simulink model "final"  (R2022b)
settings: Solver=VariableStepAuto  StartTime=0.0  StopTime=35  MaxStep=1e-4  RelTol=1e-3
libraries: simulink x8, slpidlib x5
settings Model: Creator=marco  LastModifiedBy=marco
settings SolverCC: ZeroCrossAlgorithm=Adaptive
settings DebuggingCC: MaskedZcDiagnostic=none  IgnoredZcDiagnostic=none

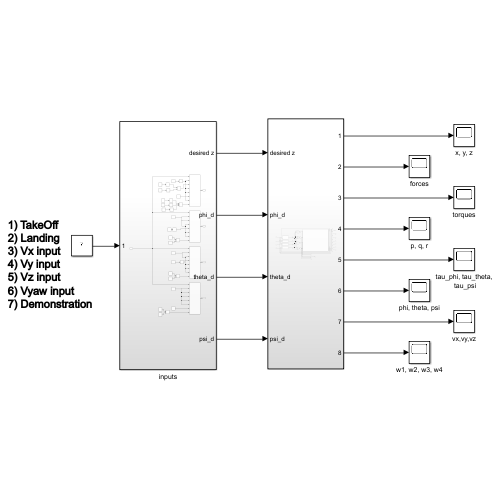
[thumbnail: Simulink's stored preview of the top-level diagram]
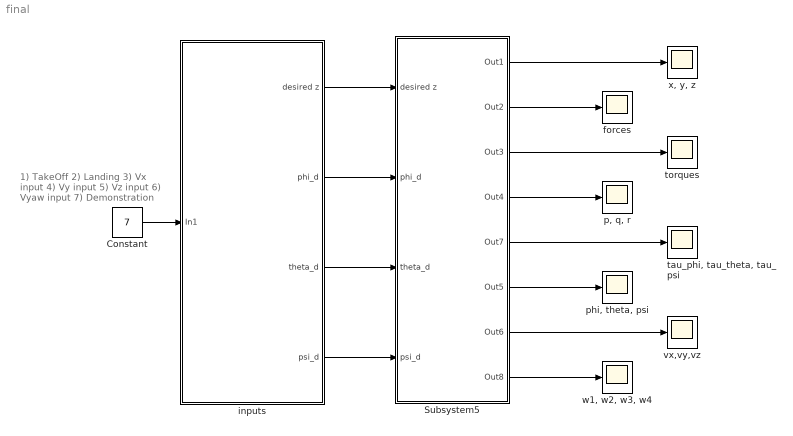
== system final ==
  note: 1) TakeOff
      | 2) Landing
      | 3) Vx input
      | 4) Vy input
      | 5) Vz input
      | 6) Vyaw input
      | 7) Demonstration
  Constant : Constant  Value=7
  Subsystem5 : Subsystem
  forces : Scope
  inputs : Subsystem
  "p, q, r" : Scope
  "phi, theta, psi" : Scope
  "tau_phi, tau_theta, tau_psi" : Scope
  torques : Scope
  vx,vy,vz : Scope
  "w1, w2, w3, w4" : Scope
  "x, y, z" : Scope
  wires:
  Constant/1 -> inputs/1(In1)
  inputs/1(desired z) -> Subsystem5/1(desired z)
  inputs/2(phi_d) -> Subsystem5/2(phi_d)
  inputs/3(theta_d) -> Subsystem5/3(theta_d)
  inputs/4(psi_d) -> Subsystem5/4(psi_d)
  Subsystem5/1(Out1) -> "x, y, z"/1
  Subsystem5/2(Out2) -> forces/1
  Subsystem5/3(Out3) -> torques/1
  Subsystem5/4(Out4) -> "p, q, r"/1
  Subsystem5/6(Out5) -> "phi, theta, psi"/1
  Subsystem5/7(Out6) -> vx,vy,vz/1
  Subsystem5/5(Out7) -> "tau_phi, tau_theta, tau_psi"/1
  Subsystem5/8(Out8) -> "w1, w2, w3, w4"/1

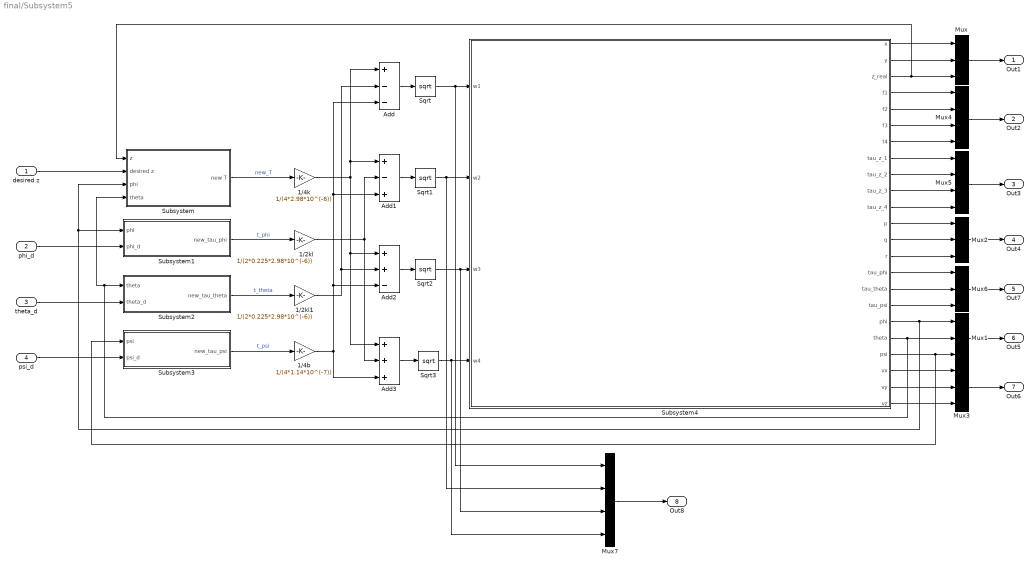
== system final/Subsystem5 ==
  desired z : Inport
  phi_d : Inport  Port=2
  theta_d : Inport  Port=3
  psi_d : Inport  Port=4
  1/2kl : Gain  Gain=1/(2*0.225*2.98*10^(-6))
  1/2kl1 : Gain  Gain=1/(2*0.225*2.98*10^(-6))
  1/4b : Gain  Gain=1/(4*1.14*10^(-7))
  1/4k : Gain  Gain=1/(4*2.98*10^(-6))
  Add : Sum  Inputs=+--
  Add1 : Sum  Inputs=+-+
  Add2 : Sum  Inputs=++-
  Add3 : Sum  Inputs=+++
  Mux{,1..3,6} (5 alike) : Mux  Inputs=3
  Mux4 : Mux
  Mux5 : Mux
  Mux7 : Mux
  Sqrt{,1..3} (4 alike) : Sqrt
  Subsystem : Subsystem
  Subsystem1 : Subsystem
  Subsystem2 : Subsystem
  Subsystem3 : Subsystem
  Subsystem4 : Subsystem
  Out1 : Outport
  Out2 : Outport  Port=2
  Out3 : Outport  Port=3
  Out4 : Outport  Port=4
  Out7 : Outport  Port=5
  Out5 : Outport  Port=6
  Out6 : Outport  Port=7
  Out8 : Outport  Port=8
  wires:
  Subsystem4/3(z_real) -> Subsystem/1(z), Mux/3
  Subsystem4/8(tau_z_1) -> Mux5/1
  1/4k/1 -> Add3/1, Add2/1, Add1/1, Add/1
  Subsystem4/19(theta) -> Subsystem2/1(theta), Subsystem/4(theta), Mux1/2
  Subsystem4/6(f3) -> Mux4/3
  Subsystem4/1(x) -> Mux/1
  Sqrt/1 -> Mux7/1, Subsystem4/1(w1)
  Mux4/1 -> Out2/1
  Subsystem4/20(psi) -> Subsystem3/1(psi), Mux1/3
  Subsystem4/4(f1) -> Mux4/1
  Subsystem4/15(tau_phi) -> Mux6/1
  1/2kl1/1 -> Add2/2, Add/2
  Subsystem4/17(tau_psi) -> Mux6/3
  Subsystem4/10(tau_z_3) -> Mux5/3
  Subsystem4/18(phi) -> Subsystem1/1(phi), Subsystem/3(phi), Mux1/1
  Subsystem4/16(tau_theta) -> Mux6/2
  Subsystem4/21(vx) -> Mux3/1
  Subsystem4/5(f2) -> Mux4/2
  Subsystem4/7(f4) -> Mux4/4
  Subsystem4/22(vy) -> Mux3/2
  Add1/1 -> Sqrt1/1
  Subsystem4/11(tau_z_4) -> Mux5/4
  Mux/1 -> Out1/1
  Sqrt1/1 -> Mux7/2, Subsystem4/2(w2)
  Mux6/1 -> Out7/1
  Subsystem3/1(new_tau_psi) -> 1/4b/1  "t_psi"
  Subsystem4/9(tau_z_2) -> Mux5/2
  1/4b/1 -> Add3/3, Add2/3, Add1/3, Add/3
  theta_d/1 -> Subsystem2/2(theta_d)
  Subsystem4/14(r) -> Mux2/3
  Subsystem/1(new T) -> 1/4k/1  "new_T"
  Subsystem2/1(new_tau_theta) -> 1/2kl1/1  "t_theta"
  Mux2/1 -> Out4/1
  Add3/1 -> Sqrt3/1
  Subsystem4/13(q) -> Mux2/2
  Subsystem4/12(p) -> Mux2/1
  Subsystem4/2(y) -> Mux/2
  1/2kl/1 -> Add3/2, Add1/2
  Sqrt3/1 -> Mux7/4, Subsystem4/4(w4)
  phi_d/1 -> Subsystem1/2(phi_d)
  Sqrt2/1 -> Mux7/3, Subsystem4/3(w3)
  Subsystem1/1(new_tau_phi) -> 1/2kl/1  "t_phi"
  Subsystem4/23(vz) -> Mux3/3
  Mux1/1 -> Out5/1
  Add2/1 -> Sqrt2/1
  Add/1 -> Sqrt/1
  Mux5/1 -> Out3/1
  desired z/1 -> Subsystem/2(desired z)
  Mux3/1 -> Out6/1
  psi_d/1 -> Subsystem3/2(psi_d)
  Mux7/1 -> Out8/1

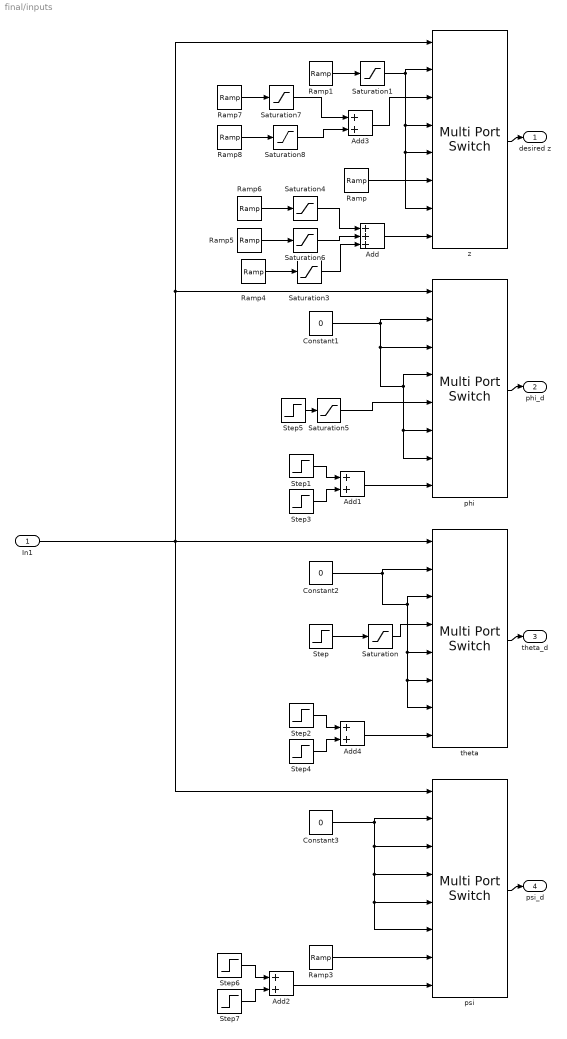
== system final/inputs ==
  In1 : Inport
  Add : Sum  Inputs=+++
  Add{1..4} (4 alike) : Sum
  Constant1 : Constant  Value=0
  Constant2 : Constant  Value=0
  Constant3 : Constant  Value=0
  Ramp : simulink/Sources/Ramp  slope=2  start=0  InitialOutput=0
  Ramp1 : simulink/Sources/Ramp  slope=1  start=0  InitialOutput=0
  Ramp3 : simulink/Sources/Ramp  slope=1  start=0  InitialOutput=0
  Ramp4 : simulink/Sources/Ramp  slope=-1  start=30  InitialOutput=0
  Ramp5 : simulink/Sources/Ramp  slope=1  start=25  InitialOutput=0
  Ramp6 : simulink/Sources/Ramp  slope=2.5  start=0  InitialOutput=0
  Ramp7 : simulink/Sources/Ramp  slope=1  start=0  InitialOutput=0
  Ramp8 : simulink/Sources/Ramp  slope=-1  start=5  InitialOutput=0
  Saturation : Saturate  UpperLimit=0.2
  Saturation{1,4,6..7} (4 alike) : Saturate  UpperLimit=1
  Saturation3 : Saturate  UpperLimit=inf  LowerLimit=-2
  Saturation5 : Saturate  UpperLimit=inf  LowerLimit=-9
  Saturation8 : Saturate  UpperLimit=1  LowerLimit=-1
  Step : Step  Time=7  After=0.05  SampleTime=0
  Step1 : Step  Time=15  After=-0.051  SampleTime=0
  Step2 : Step  Time=5  After=0.051  SampleTime=0
  Step3 : Step  Time=16  After=0.051  SampleTime=0
  Step4 : Step  Time=6  After=-0.051  SampleTime=0
  Step5 : Step  Time=5  After=-0.2  SampleTime=0
  Step6 : Step  Time=25  After=0.05  SampleTime=0
  Step7 : Step  Time=26  After=-0.05  SampleTime=0
  phi : MultiPortSwitch  Inputs=7  SaturateOnIntegerOverflow=off  InputSameDT=off
  psi : MultiPortSwitch  Inputs=7  SaturateOnIntegerOverflow=off  InputSameDT=off
  theta : MultiPortSwitch  Inputs=7  SaturateOnIntegerOverflow=off  InputSameDT=off
  z : MultiPortSwitch  Inputs=7  SaturateOnIntegerOverflow=off  InputSameDT=off
  desired z : Outport
  phi_d : Outport  Port=2
  theta_d : Outport  Port=3
  psi_d : Outport  Port=4
  wires:
  Constant2/1 -> theta/7, theta/6, theta/5, theta/3, theta/2
  Step/1 -> Saturation/1
  Constant1/1 -> phi/7, phi/6, phi/4, phi/3, phi/2
  Ramp/1 -> z/6
  Saturation1/1 -> z/7, z/5, z/4, z/2
  Constant3/1 -> psi/6, psi/5, psi/4, psi/3, psi/2
  In1/1 -> phi/1, z/1, psi/1, theta/1
  theta/1 -> theta_d/1
  Saturation/1 -> theta/4
  Ramp3/1 -> psi/7
  Ramp1/1 -> Saturation1/1
  Step5/1 -> Saturation5/1
  phi/1 -> phi_d/1
  z/1 -> desired z/1
  psi/1 -> psi_d/1
  Step4/1 -> Add4/2
  Step2/1 -> Add4/1
  Add4/1 -> theta/8
  Saturation5/1 -> phi/5
  Step1/1 -> Add1/1
  Step3/1 -> Add1/2
  Add1/1 -> phi/8
  Step6/1 -> Add2/1
  Step7/1 -> Add2/2
  Add2/1 -> psi/8
  Ramp5/1 -> Saturation6/1
  Saturation4/1 -> Add/1
  Saturation6/1 -> Add/2
  Ramp6/1 -> Saturation4/1
  Ramp4/1 -> Saturation3/1
  Saturation3/1 -> Add/3
  Add/1 -> z/8
  Saturation7/1 -> Add3/1
  Saturation8/1 -> Add3/2
  Ramp8/1 -> Saturation8/1
  Add3/1 -> z/3
  Ramp7/1 -> Saturation7/1

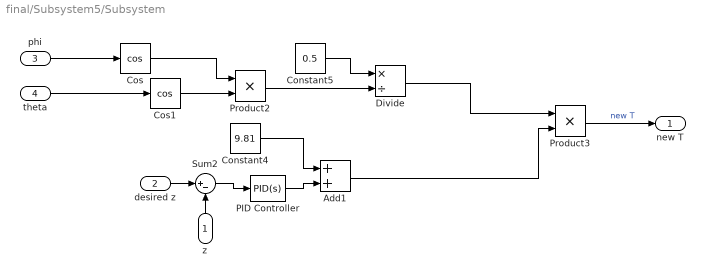
== system final/Subsystem5/Subsystem ==
  z : Inport
  desired z : Inport  Port=2
  phi : Inport  Port=3
  theta : Inport  Port=4
  Add1 : Sum
  Constant4 : Constant  Value=9.81
  Constant5 : Constant  Value=0.5
  Cos : Trigonometry  Operator=cos
  Cos1 : Trigonometry  Operator=cos
  Divide : Product  Inputs=*/
  PID Controller : slpidlib/PID Controller  Controller=PID  Form=Parallel  TimeDomain=Continuous-time  UseExternalTs=off  SampleTime=-1  IntegratorMethod=Forward Euler  FilterMethod=Forward Euler  ControllerParametersSource=internal  P=7.12587279082995  I=2.27236958573159  UseKiTs=off  D=5.19851443495758  N=56.2861343217854  UseFilter=on  TunerSelectOption=Transfer Function Based (PID Tuner App)  InitialConditionSource=internal  InitialConditionForIntegrator=0  InitialConditionForFilter=0  DifferentiatorICPrevScaledInput=0  ExternalReset=none  TrackingMode=off  Kt=1  LimitOutput=off  SatLimitsSource=internal  UpperSaturationLimit=inf  LowerSaturationLimit=-inf  LinearizeAsGain=on  AntiWindupMode=none  Kb=1  LimitIntegrator=off  UpperIntegratorSaturationLimit=inf  LowerIntegratorSaturationLimit=-inf  POutMin=[]  POutMax=[]  IOutMin=[]  IOutMax=[]  DOutMin=[]  DOutMax=[]  NOutMin=[]  NOutMax=[]  SumOutMin=[]  SumOutMax=[]  SaturationOutMin=[]  SaturationOutMax=[]  PParamMin=[]  PParamMax=[]  IParamMin=[]  IParamMax=[]  DParamMin=[]  DParamMax=[]  NParamMin=[]  NParamMax=[]  KbParamMin=[]  KbParamMax=[]  KtParamMin=[]  KtParamMax=[]  KbOutMin=[]  KbOutMax=[]  KtOutMin=[]  KtOutMax=[]  IntegratorOutMin=[]  IntegratorOutMax=[]  FilterOutMin=[]  FilterOutMax=[]  SumI1OutMin=[]  SumI1OutMax=[]  SumI2OutMin=[]  SumI2OutMax=[]  SumI3OutMin=[]  SumI3OutMax=[]  SumI4OutMin=[]  SumI4OutMax=[]  SumDOutMin=[]  SumDOutMax=[]  DifferentiatorOutMin=[]  DifferentiatorOutMax=[]  FilterDiffOutCoefMin=[]  FilterDiffOutCoefMax=[]  ReciprocalOutMin=[]  ReciprocalOutMax=[]  SumDenOutMin=[]  SumDenOutMax=[]  SumNumOutMin=[]  SumNumOutMax=[]  DivideOutMin=[]  DivideOutMax=[]  UdiffTsProdOutMin=[]  UdiffTsProdOutMax=[]  NTsProdOutMin=[]  NTsProdOutMax=[]  UintegralTsProdOutMin=[]  UintegralTsProdOutMax=[]  UngainTsProdOutMin=[]  UngainTsProdOutMax=[]  ClampingZeroOutDataTypeStr=Inherit: Inherit via back propagation  ClampingZeroOutMin=[]  ClampingZeroOutMax=[]  FilterDenConstantOutDataTypeStr=Inherit: Inherit via back propagation  FilterDenConstantOutMin=[]  FilterDenConstantOutMax=[]  PCopyOutDataTypeStr=Inherit: Inherit via back propagation  PCopyOutMin=[]  PCopyOutMax=[]  NCopyOutDataTypeStr=Inherit: Inherit via back propagation  NCopyOutMin=[]  NCopyOutMax=[]  IntegratorContinuousStateAttributes=''  IntegratorStateMustResolveToSignalObject=off  IntegratorRTWStateStorageClass=Auto  FilterContinuousStateAttributes=''  FilterStateMustResolveToSignalObject=off  FilterRTWStateStorageClass=Auto  ParallelPVariant=InternalParameters  IdealPVariant=Disabled  IVariant=InternalParameters  DVariant=InternalParameters  IntegratorVariant=Continuous  SatVariant=Disabled  AWVariant=Passthrough  PCopyVariant=Disabled  TRVariant=Disabled  FdbkBlocksVariant=Forward  IdealPFdbkVariant=Disabled  SatFdbkVariant=Disabled  DerivativeFilterVariant=ContFilter  NVariant=InternalParameters  NCopyVariant=Disabled  FilterICVariant=InternalICsFilter  IntegratorICVariant=InternalICs  ExternalResetVariant=Disabled  TRSumVariant=Passthrough  SumFdbkVariant=Disabled  SumVariant=Sum_PID  TsampFilterVariant=InternalTs  TsampNgainVariant=Passthrough  TsampIntegralVariant=Passthrough  ExternalSaturationOutDataTypeStr=Inherit: Same as second input
  Product2 : Product
  Product3 : Product
  Sum2 : Sum  Inputs=|+-
  new T : Outport
  wires:
  Constant4/1 -> Add1/1
  Product2/1 -> Divide/2
  Divide/1 -> Product3/1
  Product3/1 -> new T/1  "new T"
  Cos/1 -> Product2/1
  phi/1 -> Cos/1
  Cos1/1 -> Product2/2
  z/1 -> Sum2/2
  Constant5/1 -> Divide/1
  theta/1 -> Cos1/1
  desired z/1 -> Sum2/1
  Sum2/1 -> PID Controller/1
  PID Controller/1 -> Add1/2
  Add1/1 -> Product3/2

== system final/Subsystem5/Subsystem1 ==
  phi : Inport
  phi_d : Inport  Port=2
  Ix : Gain  Gain=4.856*10^(-3)
  PID Controller : slpidlib/PID Controller  Controller=PID  Form=Parallel  TimeDomain=Continuous-time  UseExternalTs=off  SampleTime=-1  IntegratorMethod=Forward Euler  FilterMethod=Forward Euler  ControllerParametersSource=internal  P=7.44259083470397  I=2.2059084504827  UseKiTs=off  D=6.16600811387227  N=34.5297262058638  UseFilter=on  TunerSelectOption=Transfer Function Based (PID Tuner App)  InitialConditionSource=internal  InitialConditionForIntegrator=0  InitialConditionForFilter=0  DifferentiatorICPrevScaledInput=0  ExternalReset=none  TrackingMode=off  Kt=1  LimitOutput=off  SatLimitsSource=internal  UpperSaturationLimit=inf  LowerSaturationLimit=-inf  LinearizeAsGain=on  AntiWindupMode=none  Kb=1  LimitIntegrator=off  UpperIntegratorSaturationLimit=inf  LowerIntegratorSaturationLimit=-inf  POutMin=[]  POutMax=[]  IOutMin=[]  IOutMax=[]  DOutMin=[]  DOutMax=[]  NOutMin=[]  NOutMax=[]  SumOutMin=[]  SumOutMax=[]  SaturationOutMin=[]  SaturationOutMax=[]  PParamMin=[]  PParamMax=[]  IParamMin=[]  IParamMax=[]  DParamMin=[]  DParamMax=[]  NParamMin=[]  NParamMax=[]  KbParamMin=[]  KbParamMax=[]  KtParamMin=[]  KtParamMax=[]  KbOutMin=[]  KbOutMax=[]  KtOutMin=[]  KtOutMax=[]  IntegratorOutMin=[]  IntegratorOutMax=[]  FilterOutMin=[]  FilterOutMax=[]  SumI1OutMin=[]  SumI1OutMax=[]  SumI2OutMin=[]  SumI2OutMax=[]  SumI3OutMin=[]  SumI3OutMax=[]  SumI4OutMin=[]  SumI4OutMax=[]  SumDOutMin=[]  SumDOutMax=[]  DifferentiatorOutMin=[]  DifferentiatorOutMax=[]  FilterDiffOutCoefMin=[]  FilterDiffOutCoefMax=[]  ReciprocalOutMin=[]  ReciprocalOutMax=[]  SumDenOutMin=[]  SumDenOutMax=[]  SumNumOutMin=[]  SumNumOutMax=[]  DivideOutMin=[]  DivideOutMax=[]  UdiffTsProdOutMin=[]  UdiffTsProdOutMax=[]  NTsProdOutMin=[]  NTsProdOutMax=[]  UintegralTsProdOutMin=[]  UintegralTsProdOutMax=[]  UngainTsProdOutMin=[]  UngainTsProdOutMax=[]  ClampingZeroOutDataTypeStr=Inherit: Inherit via back propagation  ClampingZeroOutMin=[]  ClampingZeroOutMax=[]  FilterDenConstantOutDataTypeStr=Inherit: Inherit via back propagation  FilterDenConstantOutMin=[]  FilterDenConstantOutMax=[]  PCopyOutDataTypeStr=Inherit: Inherit via back propagation  PCopyOutMin=[]  PCopyOutMax=[]  NCopyOutDataTypeStr=Inherit: Inherit via back propagation  NCopyOutMin=[]  NCopyOutMax=[]  IntegratorContinuousStateAttributes=''  IntegratorStateMustResolveToSignalObject=off  IntegratorRTWStateStorageClass=Auto  FilterContinuousStateAttributes=''  FilterStateMustResolveToSignalObject=off  FilterRTWStateStorageClass=Auto  ParallelPVariant=InternalParameters  IdealPVariant=Disabled  IVariant=InternalParameters  DVariant=InternalParameters  IntegratorVariant=Continuous  SatVariant=Disabled  AWVariant=Passthrough  PCopyVariant=Disabled  TRVariant=Disabled  FdbkBlocksVariant=Forward  IdealPFdbkVariant=Disabled  SatFdbkVariant=Disabled  DerivativeFilterVariant=ContFilter  NVariant=InternalParameters  NCopyVariant=Disabled  FilterICVariant=InternalICsFilter  IntegratorICVariant=InternalICs  ExternalResetVariant=Disabled  TRSumVariant=Passthrough  SumFdbkVariant=Disabled  SumVariant=Sum_PID  TsampFilterVariant=InternalTs  TsampNgainVariant=Passthrough  TsampIntegralVariant=Passthrough  ExternalSaturationOutDataTypeStr=Inherit: Same as second input
  Sum2 : Sum  Inputs=|+-
  new_tau_phi : Outport
  wires:
  phi_d/1 -> Sum2/1
  phi/1 -> Sum2/2
  Ix/1 -> new_tau_phi/1
  Sum2/1 -> PID Controller/1
  PID Controller/1 -> Ix/1

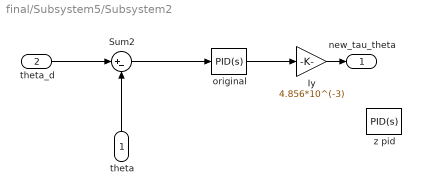
== system final/Subsystem5/Subsystem2 ==
  theta : Inport
  theta_d : Inport  Port=2
  Iy : Gain  Gain=4.856*10^(-3)
  Sum2 : Sum  Inputs=|+-
  original : slpidlib/PID Controller  Controller=PID  Form=Parallel  TimeDomain=Continuous-time  UseExternalTs=off  SampleTime=-1  IntegratorMethod=Forward Euler  FilterMethod=Forward Euler  ControllerParametersSource=internal  P=7.44259083470397  I=2.2059084504827  UseKiTs=off  D=6.16600811387227  N=34.5297262058638  UseFilter=on  TunerSelectOption=Transfer Function Based (PID Tuner App)  InitialConditionSource=internal  InitialConditionForIntegrator=0  InitialConditionForFilter=0  DifferentiatorICPrevScaledInput=0  ExternalReset=none  TrackingMode=off  Kt=1  LimitOutput=off  SatLimitsSource=internal  UpperSaturationLimit=inf  LowerSaturationLimit=-inf  LinearizeAsGain=on  AntiWindupMode=none  Kb=1  LimitIntegrator=off  UpperIntegratorSaturationLimit=inf  LowerIntegratorSaturationLimit=-inf  POutMin=[]  POutMax=[]  IOutMin=[]  IOutMax=[]  DOutMin=[]  DOutMax=[]  NOutMin=[]  NOutMax=[]  SumOutMin=[]  SumOutMax=[]  SaturationOutMin=[]  SaturationOutMax=[]  PParamMin=[]  PParamMax=[]  IParamMin=[]  IParamMax=[]  DParamMin=[]  DParamMax=[]  NParamMin=[]  NParamMax=[]  KbParamMin=[]  KbParamMax=[]  KtParamMin=[]  KtParamMax=[]  KbOutMin=[]  KbOutMax=[]  KtOutMin=[]  KtOutMax=[]  IntegratorOutMin=[]  IntegratorOutMax=[]  FilterOutMin=[]  FilterOutMax=[]  SumI1OutMin=[]  SumI1OutMax=[]  SumI2OutMin=[]  SumI2OutMax=[]  SumI3OutMin=[]  SumI3OutMax=[]  SumI4OutMin=[]  SumI4OutMax=[]  SumDOutMin=[]  SumDOutMax=[]  DifferentiatorOutMin=[]  DifferentiatorOutMax=[]  FilterDiffOutCoefMin=[]  FilterDiffOutCoefMax=[]  ReciprocalOutMin=[]  ReciprocalOutMax=[]  SumDenOutMin=[]  SumDenOutMax=[]  SumNumOutMin=[]  SumNumOutMax=[]  DivideOutMin=[]  DivideOutMax=[]  UdiffTsProdOutMin=[]  UdiffTsProdOutMax=[]  NTsProdOutMin=[]  NTsProdOutMax=[]  UintegralTsProdOutMin=[]  UintegralTsProdOutMax=[]  UngainTsProdOutMin=[]  UngainTsProdOutMax=[]  ClampingZeroOutDataTypeStr=Inherit: Inherit via back propagation  ClampingZeroOutMin=[]  ClampingZeroOutMax=[]  FilterDenConstantOutDataTypeStr=Inherit: Inherit via back propagation  FilterDenConstantOutMin=[]  FilterDenConstantOutMax=[]  PCopyOutDataTypeStr=Inherit: Inherit via back propagation  PCopyOutMin=[]  PCopyOutMax=[]  NCopyOutDataTypeStr=Inherit: Inherit via back propagation  NCopyOutMin=[]  NCopyOutMax=[]  IntegratorContinuousStateAttributes=''  IntegratorStateMustResolveToSignalObject=off  IntegratorRTWStateStorageClass=Auto  FilterContinuousStateAttributes=''  FilterStateMustResolveToSignalObject=off  FilterRTWStateStorageClass=Auto  ParallelPVariant=InternalParameters  IdealPVariant=Disabled  IVariant=InternalParameters  DVariant=InternalParameters  IntegratorVariant=Continuous  SatVariant=Disabled  AWVariant=Passthrough  PCopyVariant=Disabled  TRVariant=Disabled  FdbkBlocksVariant=Forward  IdealPFdbkVariant=Disabled  SatFdbkVariant=Disabled  DerivativeFilterVariant=ContFilter  NVariant=InternalParameters  NCopyVariant=Disabled  FilterICVariant=InternalICsFilter  IntegratorICVariant=InternalICs  ExternalResetVariant=Disabled  TRSumVariant=Passthrough  SumFdbkVariant=Disabled  SumVariant=Sum_PID  TsampFilterVariant=InternalTs  TsampNgainVariant=Passthrough  TsampIntegralVariant=Passthrough  ExternalSaturationOutDataTypeStr=Inherit: Same as second input
  z pid : slpidlib/PID Controller  Controller=PID  Form=Parallel  TimeDomain=Continuous-time  UseExternalTs=off  SampleTime=-1  IntegratorMethod=Forward Euler  FilterMethod=Forward Euler  ControllerParametersSource=internal  P=7.12587279082995  I=2.27236958573159  UseKiTs=off  D=5.19851443495758  N=56.2861343217854  UseFilter=on  TunerSelectOption=Transfer Function Based (PID Tuner App)  InitialConditionSource=internal  InitialConditionForIntegrator=0  InitialConditionForFilter=0  DifferentiatorICPrevScaledInput=0  ExternalReset=none  TrackingMode=off  Kt=1  LimitOutput=off  SatLimitsSource=internal  UpperSaturationLimit=inf  LowerSaturationLimit=-inf  LinearizeAsGain=on  AntiWindupMode=none  Kb=1  LimitIntegrator=off  UpperIntegratorSaturationLimit=inf  LowerIntegratorSaturationLimit=-inf  POutMin=[]  POutMax=[]  IOutMin=[]  IOutMax=[]  DOutMin=[]  DOutMax=[]  NOutMin=[]  NOutMax=[]  SumOutMin=[]  SumOutMax=[]  SaturationOutMin=[]  SaturationOutMax=[]  PParamMin=[]  PParamMax=[]  IParamMin=[]  IParamMax=[]  DParamMin=[]  DParamMax=[]  NParamMin=[]  NParamMax=[]  KbParamMin=[]  KbParamMax=[]  KtParamMin=[]  KtParamMax=[]  KbOutMin=[]  KbOutMax=[]  KtOutMin=[]  KtOutMax=[]  IntegratorOutMin=[]  IntegratorOutMax=[]  FilterOutMin=[]  FilterOutMax=[]  SumI1OutMin=[]  SumI1OutMax=[]  SumI2OutMin=[]  SumI2OutMax=[]  SumI3OutMin=[]  SumI3OutMax=[]  SumI4OutMin=[]  SumI4OutMax=[]  SumDOutMin=[]  SumDOutMax=[]  DifferentiatorOutMin=[]  DifferentiatorOutMax=[]  FilterDiffOutCoefMin=[]  FilterDiffOutCoefMax=[]  ReciprocalOutMin=[]  ReciprocalOutMax=[]  SumDenOutMin=[]  SumDenOutMax=[]  SumNumOutMin=[]  SumNumOutMax=[]  DivideOutMin=[]  DivideOutMax=[]  UdiffTsProdOutMin=[]  UdiffTsProdOutMax=[]  NTsProdOutMin=[]  NTsProdOutMax=[]  UintegralTsProdOutMin=[]  UintegralTsProdOutMax=[]  UngainTsProdOutMin=[]  UngainTsProdOutMax=[]  ClampingZeroOutDataTypeStr=Inherit: Inherit via back propagation  ClampingZeroOutMin=[]  ClampingZeroOutMax=[]  FilterDenConstantOutDataTypeStr=Inherit: Inherit via back propagation  FilterDenConstantOutMin=[]  FilterDenConstantOutMax=[]  PCopyOutDataTypeStr=Inherit: Inherit via back propagation  PCopyOutMin=[]  PCopyOutMax=[]  NCopyOutDataTypeStr=Inherit: Inherit via back propagation  NCopyOutMin=[]  NCopyOutMax=[]  IntegratorContinuousStateAttributes=''  IntegratorStateMustResolveToSignalObject=off  IntegratorRTWStateStorageClass=Auto  FilterContinuousStateAttributes=''  FilterStateMustResolveToSignalObject=off  FilterRTWStateStorageClass=Auto  ParallelPVariant=InternalParameters  IdealPVariant=Disabled  IVariant=InternalParameters  DVariant=InternalParameters  IntegratorVariant=Continuous  SatVariant=Disabled  AWVariant=Passthrough  PCopyVariant=Disabled  TRVariant=Disabled  FdbkBlocksVariant=Forward  IdealPFdbkVariant=Disabled  SatFdbkVariant=Disabled  DerivativeFilterVariant=ContFilter  NVariant=InternalParameters  NCopyVariant=Disabled  FilterICVariant=InternalICsFilter  IntegratorICVariant=InternalICs  ExternalResetVariant=Disabled  TRSumVariant=Passthrough  SumFdbkVariant=Disabled  SumVariant=Sum_PID  TsampFilterVariant=InternalTs  TsampNgainVariant=Passthrough  TsampIntegralVariant=Passthrough  ExternalSaturationOutDataTypeStr=Inherit: Same as second input
  new_tau_theta : Outport
  wires:
  theta_d/1 -> Sum2/1
  theta/1 -> Sum2/2
  Iy/1 -> new_tau_theta/1
  original/1 -> Iy/1
  Sum2/1 -> original/1

== system final/Subsystem5/Subsystem3 ==
  psi : Inport
  psi_d : Inport  Port=2
  Iz : Gain  Gain=8.801*10^(-3)
  PID Controller1 : slpidlib/PID Controller  Controller=PID  Form=Parallel  TimeDomain=Continuous-time  UseExternalTs=off  SampleTime=-1  IntegratorMethod=Forward Euler  FilterMethod=Forward Euler  ControllerParametersSource=internal  P=19.126699464281  I=9.13192175933972  UseKiTs=off  D=9.75332765558192  N=36.46824066771  UseFilter=on  TunerSelectOption=Transfer Function Based (PID Tuner App)  InitialConditionSource=internal  InitialConditionForIntegrator=0  InitialConditionForFilter=0  DifferentiatorICPrevScaledInput=0  ExternalReset=none  TrackingMode=off  Kt=1  LimitOutput=off  SatLimitsSource=internal  UpperSaturationLimit=inf  LowerSaturationLimit=-inf  LinearizeAsGain=on  AntiWindupMode=none  Kb=1  LimitIntegrator=off  UpperIntegratorSaturationLimit=inf  LowerIntegratorSaturationLimit=-inf  POutMin=[]  POutMax=[]  IOutMin=[]  IOutMax=[]  DOutMin=[]  DOutMax=[]  NOutMin=[]  NOutMax=[]  SumOutMin=[]  SumOutMax=[]  SaturationOutMin=[]  SaturationOutMax=[]  PParamMin=[]  PParamMax=[]  IParamMin=[]  IParamMax=[]  DParamMin=[]  DParamMax=[]  NParamMin=[]  NParamMax=[]  KbParamMin=[]  KbParamMax=[]  KtParamMin=[]  KtParamMax=[]  KbOutMin=[]  KbOutMax=[]  KtOutMin=[]  KtOutMax=[]  IntegratorOutMin=[]  IntegratorOutMax=[]  FilterOutMin=[]  FilterOutMax=[]  SumI1OutMin=[]  SumI1OutMax=[]  SumI2OutMin=[]  SumI2OutMax=[]  SumI3OutMin=[]  SumI3OutMax=[]  SumI4OutMin=[]  SumI4OutMax=[]  SumDOutMin=[]  SumDOutMax=[]  DifferentiatorOutMin=[]  DifferentiatorOutMax=[]  FilterDiffOutCoefMin=[]  FilterDiffOutCoefMax=[]  ReciprocalOutMin=[]  ReciprocalOutMax=[]  SumDenOutMin=[]  SumDenOutMax=[]  SumNumOutMin=[]  SumNumOutMax=[]  DivideOutMin=[]  DivideOutMax=[]  UdiffTsProdOutMin=[]  UdiffTsProdOutMax=[]  NTsProdOutMin=[]  NTsProdOutMax=[]  UintegralTsProdOutMin=[]  UintegralTsProdOutMax=[]  UngainTsProdOutMin=[]  UngainTsProdOutMax=[]  ClampingZeroOutDataTypeStr=Inherit: Inherit via back propagation  ClampingZeroOutMin=[]  ClampingZeroOutMax=[]  FilterDenConstantOutDataTypeStr=Inherit: Inherit via back propagation  FilterDenConstantOutMin=[]  FilterDenConstantOutMax=[]  PCopyOutDataTypeStr=Inherit: Inherit via back propagation  PCopyOutMin=[]  PCopyOutMax=[]  NCopyOutDataTypeStr=Inherit: Inherit via back propagation  NCopyOutMin=[]  NCopyOutMax=[]  IntegratorContinuousStateAttributes=''  IntegratorStateMustResolveToSignalObject=off  IntegratorRTWStateStorageClass=Auto  FilterContinuousStateAttributes=''  FilterStateMustResolveToSignalObject=off  FilterRTWStateStorageClass=Auto  ParallelPVariant=InternalParameters  IdealPVariant=Disabled  IVariant=InternalParameters  DVariant=InternalParameters  IntegratorVariant=Continuous  SatVariant=Disabled  AWVariant=Passthrough  PCopyVariant=Disabled  TRVariant=Disabled  FdbkBlocksVariant=Forward  IdealPFdbkVariant=Disabled  SatFdbkVariant=Disabled  DerivativeFilterVariant=ContFilter  NVariant=InternalParameters  NCopyVariant=Disabled  FilterICVariant=InternalICsFilter  IntegratorICVariant=InternalICs  ExternalResetVariant=Disabled  TRSumVariant=Passthrough  SumFdbkVariant=Disabled  SumVariant=Sum_PID  TsampFilterVariant=InternalTs  TsampNgainVariant=Passthrough  TsampIntegralVariant=Passthrough  ExternalSaturationOutDataTypeStr=Inherit: Same as second input
  Sum2 : Sum  Inputs=|+-
  new_tau_psi : Outport
  wires:
  psi_d/1 -> Sum2/1
  psi/1 -> Sum2/2
  Iz/1 -> new_tau_psi/1
  PID Controller1/1 -> Iz/1
  Sum2/1 -> PID Controller1/1

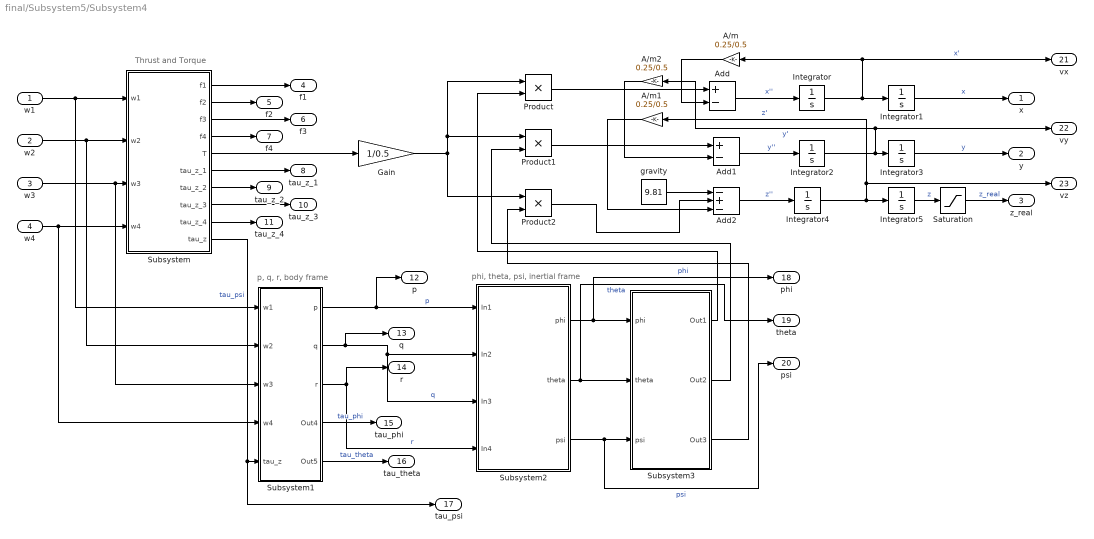
== system final/Subsystem5/Subsystem4 ==
  note: phi, theta, psi, inertial frame
  note: p, q, r, body frame
  note: Thrust and Torque
  w1 : Inport
  w2 : Inport  Port=2
  w3 : Inport  Port=3
  w4 : Inport  Port=4
  A/m : Gain  Gain=0.25/0.5
  A/m1 : Gain  Gain=0.25/0.5
  A/m2 : Gain  Gain=0.25/0.5
  Add : Sum  Inputs=+-
  Add1 : Sum  Inputs=+-
  Add2 : Sum  Inputs=-+-
  Gain : Gain  Gain=1/0.5
  Integrator{,1..5} (6 alike) : Integrator
  Product : Product
  Product1 : Product
  Product2 : Product
  Saturation : Saturate  UpperLimit=inf  LowerLimit=0
  Subsystem : Subsystem
  Subsystem1 : Subsystem  mask{Ix=4.856*10^(-3), Iy=4.856*10^(-3), Iz=8.801*10^(-3), Ir=0.005, l=0.225, k=2.98*10^(-6)}
      mask prompts: Ix "inertia on x"; Iy "inertia on y"; Iz "inertia on z"; Ir "radial inertia"; l "arm distance"; k "lift coefficient"
  Subsystem2 : Subsystem
  Subsystem3 : Subsystem
  gravity : Constant  Value=9.81
  x : Outport
  y : Outport  Port=2
  z_real : Outport  Port=3
  f1 : Outport  Port=4
  f2 : Outport  Port=5
  f3 : Outport  Port=6
  f4 : Outport  Port=7
  tau_z_1 : Outport  Port=8
  tau_z_2 : Outport  Port=9
  tau_z_3 : Outport  Port=10
  tau_z_4 : Outport  Port=11
  p : Outport  Port=12
  q : Outport  Port=13
  r : Outport  Port=14
  tau_phi : Outport  Port=15
  tau_theta : Outport  Port=16
  tau_psi : Outport  Port=17
  phi : Outport  Port=18
  theta : Outport  Port=19
  psi : Outport  Port=20
  vx : Outport  Port=21
  vy : Outport  Port=22
  vz : Outport  Port=23
  wires:
  A/m/1 -> Add/2
  Integrator3/1 -> y/1  "y"
  Subsystem2/1(phi) -> phi/1, Subsystem3/1(phi)  "phi"
  Subsystem1/1(p) -> p/1, Subsystem2/1(In1)  "p"
  Subsystem1/2(q) -> q/1, Subsystem2/2(In2), Subsystem2/3(In3)  "q"
  Subsystem2/2(theta) -> theta/1, Subsystem3/2(theta)  "theta"
  Add/1 -> Integrator/1  "x''"
  Subsystem3/2(Out2) -> Product1/2
  Subsystem3/1(Out1) -> Product/2
  Integrator2/1 -> Integrator3/1, A/m2/1, vy/1  "y'"
  Gain/1 -> Product/1, Product1/1, Product2/1
  Add1/1 -> Integrator2/1  "y''"
  Integrator/1 -> vx/1, A/m/1, Integrator1/1  "x'"
  Subsystem1/4(Out4) -> tau_phi/1  "tau_phi"
  Subsystem1/5(Out5) -> tau_theta/1  "tau_theta"
  gravity/1 -> Add2/1
  A/m2/1 -> Add1/2
  Subsystem/4(f4) -> f4/1
  Integrator4/1 -> A/m1/1, vz/1, Integrator5/1  "z'"
  Subsystem/8(tau_z_3) -> tau_z_3/1
  Product/1 -> Add/1
  Subsystem1/3(r) -> r/1, Subsystem2/4(In4)  "r"
  Subsystem/3(f3) -> f3/1
  w1/1 -> Subsystem1/1(w1), Subsystem/1(w1)
  w2/1 -> Subsystem1/2(w2), Subsystem/2(w2)
  w3/1 -> Subsystem1/3(w3), Subsystem/3(w3)
  Subsystem2/3(psi) -> psi/1, Subsystem3/3(psi)  "psi"
  w4/1 -> Subsystem1/4(w4), Subsystem/4(w4)
  Add2/1 -> Integrator4/1  "z''"
  Product2/1 -> Add2/2
  Subsystem/10(tau_z) -> tau_psi/1, Subsystem1/5(tau_z)  "tau_psi"
  Integrator1/1 -> x/1  "x"
  Integrator5/1 -> Saturation/1  "z"
  Subsystem3/3(Out3) -> Product2/2
  Product1/1 -> Add1/1
  A/m1/1 -> Add2/3
  Subsystem/5(T) -> Gain/1
  Subsystem/7(tau_z_2) -> tau_z_2/1
  Saturation/1 -> z_real/1  "z_real"
  Subsystem/6(tau_z_1) -> tau_z_1/1
  Subsystem/2(f2) -> f2/1
  Subsystem/9(tau_z_4) -> tau_z_4/1
  Subsystem/1(f1) -> f1/1

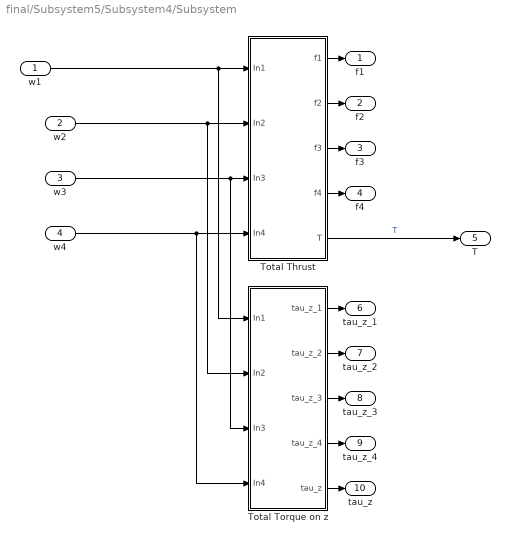
== system final/Subsystem5/Subsystem4/Subsystem ==
  w1 : Inport
  w2 : Inport  Port=2
  w3 : Inport  Port=3
  w4 : Inport  Port=4
  Total Thrust : Subsystem  mask{k=2.98*10^(-6)}
      mask prompts: k "Lift Coefficient"
  Total Torque on z : Subsystem  mask{b=1.14*10^(-7), I_m=3.357*10^(-5)}
      mask prompts: b "Drag Coefficient"; I_m "Inertia of the rotor"
  f1 : Outport
  f2 : Outport  Port=2
  f3 : Outport  Port=3
  f4 : Outport  Port=4
  T : Outport  Port=5
  tau_z_1 : Outport  Port=6
  tau_z_2 : Outport  Port=7
  tau_z_3 : Outport  Port=8
  tau_z_4 : Outport  Port=9
  tau_z : Outport  Port=10
  wires:
  Total Torque on z/5(tau_z) -> tau_z/1
  Total Thrust/5(T) -> T/1  "T"
  w4/1 -> Total Torque on z/4(In4), Total Thrust/4(In4)
  Total Torque on z/4(tau_z_4) -> tau_z_4/1
  w1/1 -> Total Torque on z/1(In1), Total Thrust/1(In1)
  w3/1 -> Total Torque on z/3(In3), Total Thrust/3(In3)
  Total Thrust/4(f4) -> f4/1
  Total Thrust/1(f1) -> f1/1
  w2/1 -> Total Torque on z/2(In2), Total Thrust/2(In2)
  Total Torque on z/1(tau_z_1) -> tau_z_1/1
  Total Torque on z/2(tau_z_2) -> tau_z_2/1
  Total Torque on z/3(tau_z_3) -> tau_z_3/1
  Total Thrust/3(f3) -> f3/1
  Total Thrust/2(f2) -> f2/1

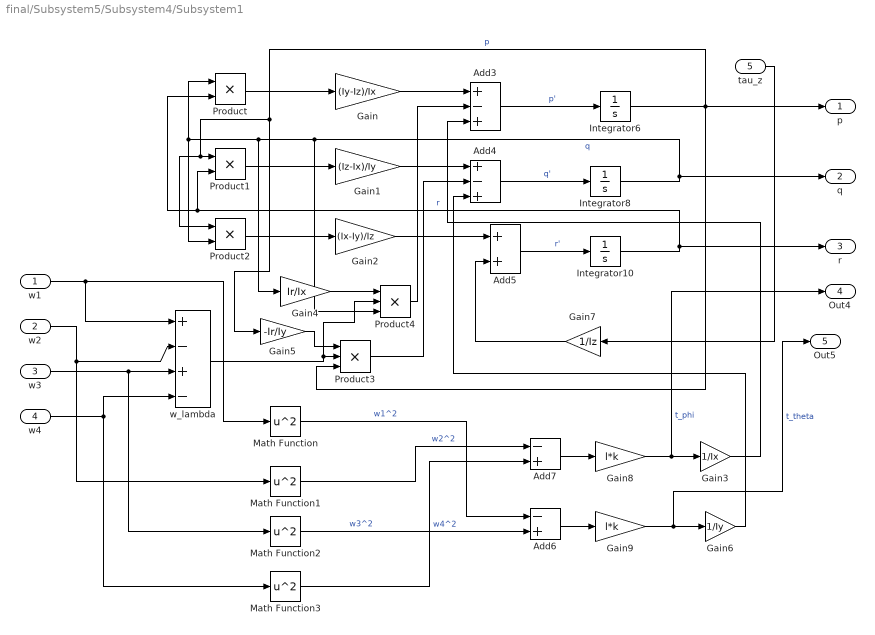
== system final/Subsystem5/Subsystem4/Subsystem1 ==
  w1 : Inport
  w2 : Inport  Port=2
  w3 : Inport  Port=3
  w4 : Inport  Port=4
  tau_z : Inport  Port=5
  Add3 : Sum  Inputs=+-+
  Add4 : Sum  Inputs=+-+
  Add5 : Sum
  Add6 : Sum  Inputs=-+
  Add7 : Sum  Inputs=-+
  Gain : Gain  Gain=(Iy-Iz)/Ix
  Gain1 : Gain  Gain=(Iz-Ix)/Iy
  Gain2 : Gain  Gain=(Ix-Iy)/Iz
  Gain3 : Gain  Gain=1/Ix
  Gain4 : Gain  Gain=Ir/Ix
  Gain5 : Gain  Gain=-Ir/Iy
  Gain6 : Gain  Gain=1/Iy
  Gain7 : Gain  Gain=1/Iz
  Gain8 : Gain  Gain=l*k
  Gain9 : Gain  Gain=l*k
  Integrator10 : Integrator
  Integrator6 : Integrator
  Integrator8 : Integrator
  Math Function{,1..3} (4 alike) : Math  Operator=square
  Product : Product
  Product1 : Product
  Product2 : Product
  Product3 : Product  Inputs=3
  Product4 : Product  Inputs=3
  w_lambda : Sum  Inputs=+-+-
  p : Outport
  q : Outport  Port=2
  r : Outport  Port=3
  Out4 : Outport  Port=4
  Out5 : Outport  Port=5
  wires:
  Add3/1 -> Integrator6/1  "p'"
  Integrator8/1 -> Product2/2, Product/1, Gain4/1, Product4/3, q/1  "q"
  Product1/1 -> Gain1/1
  w4/1 -> Math Function3/1, w_lambda/4
  w2/1 -> Math Function1/1, w_lambda/2
  Gain6/1 -> Add4/3
  Gain8/1 -> Out4/1, Gain3/1  "t_phi"
  Add5/1 -> Integrator10/1  "r'"
  Gain/1 -> Add3/1
  Integrator6/1 -> Product3/3, p/1, Gain5/1, Product2/1, Product1/1  "p"
  w_lambda/1 -> Product4/2, Product3/2
  Integrator10/1 -> r/1, Product1/2, Product/2  "r"
  Math Function1/1 -> Add7/1  "w2^2"
  Gain9/1 -> Out5/1, Gain6/1  "t_theta"
  Math Function3/1 -> Add7/2  "w4^2"
  Math Function2/1 -> Add6/2  "w3^2"
  w3/1 -> Math Function2/1, w_lambda/3
  Gain7/1 -> Add5/2
  w1/1 -> Math Function/1, w_lambda/1
  Gain3/1 -> Add3/3
  Product/1 -> Gain/1
  Math Function/1 -> Add6/1  "w1^2"
  Gain5/1 -> Product3/1
  Add7/1 -> Gain8/1
  Add6/1 -> Gain9/1
  Gain1/1 -> Add4/1
  Add4/1 -> Integrator8/1  "q'"
  Product4/1 -> Add3/2
  Product2/1 -> Gain2/1
  Gain2/1 -> Add5/1
  Product3/1 -> Add4/2
  Gain4/1 -> Product4/1
  tau_z/1 -> Gain7/1

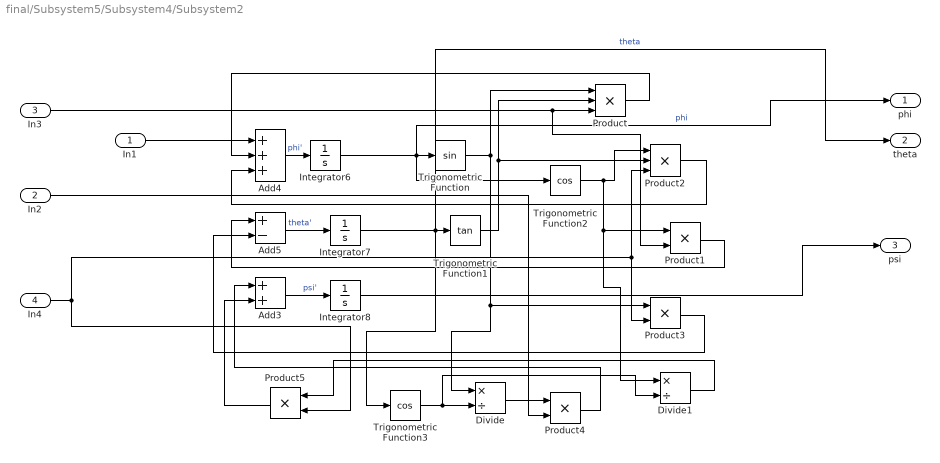
== system final/Subsystem5/Subsystem4/Subsystem2 ==
  In1 : Inport
  In2 : Inport  Port=2
  In3 : Inport  Port=3
  In4 : Inport  Port=4
  Add3 : Sum
  Add4 : Sum  Inputs=+++
  Add5 : Sum  Inputs=+-
  Divide : Product  Inputs=*/
  Divide1 : Product  Inputs=*/
  Integrator6 : Integrator
  Integrator7 : Integrator
  Integrator8 : Integrator
  Product : Product  Inputs=3
  Product{1,3..5} (4 alike) : Product
  Product2 : Product  Inputs=3
  Trigonometric Function : Trigonometry
  Trigonometric Function1 : Trigonometry  Operator=tan
  Trigonometric Function2 : Trigonometry  Operator=cos
  Trigonometric Function3 : Trigonometry  Operator=cos
  phi : Outport
  theta : Outport  Port=2
  psi : Outport  Port=3
  wires:
  Product1/1 -> Add5/1
  Add4/1 -> Integrator6/1  "phi'"
  Trigonometric Function3/1 -> Divide1/2, Divide/2
  Trigonometric Function/1 -> Divide/1, Product3/1, Product/1
  Product5/1 -> Add3/2
  Integrator7/1 -> Trigonometric Function3/1, Trigonometric Function1/1, theta/1  "theta"
  Add5/1 -> Integrator7/1  "theta'"
  Integrator6/1 -> Trigonometric Function2/1, Trigonometric Function/1, phi/1  "phi"
  Trigonometric Function2/1 -> Divide1/1, Product1/1, Product2/1
  Add3/1 -> Integrator8/1  "psi'"
  In4/1 -> Product3/2, Product2/3, Product5/2
  Product3/1 -> Add5/2
  Divide/1 -> Product4/1
  Divide1/1 -> Product5/1
  Trigonometric Function1/1 -> Product/2, Product2/2
  Product4/1 -> Add3/1
  In3/1 -> Product1/2, Product/3
  Product2/1 -> Add4/3
  Product/1 -> Add4/2
  In1/1 -> Add4/1
  In2/1 -> Product4/2
  Integrator8/1 -> psi/1

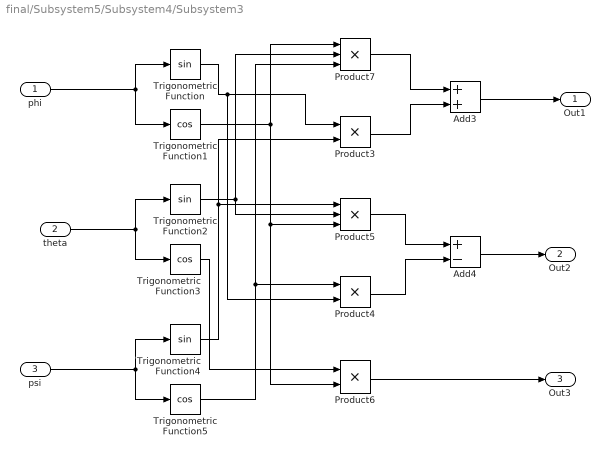
== system final/Subsystem5/Subsystem4/Subsystem3 ==
  phi : Inport
  theta : Inport  Port=2
  psi : Inport  Port=3
  Add3 : Sum
  Add4 : Sum  Inputs=+-
  Product3 : Product
  Product4 : Product
  Product5 : Product  Inputs=3
  Product6 : Product
  Product7 : Product  Inputs=3
  Trigonometric Function : Trigonometry
  Trigonometric Function1 : Trigonometry  Operator=cos
  Trigonometric Function2 : Trigonometry
  Trigonometric Function3 : Trigonometry  Operator=cos
  Trigonometric Function4 : Trigonometry
  Trigonometric Function5 : Trigonometry  Operator=cos
  Out1 : Outport
  Out2 : Outport  Port=2
  Out3 : Outport  Port=3
  wires:
  psi/1 -> Trigonometric Function5/1, Trigonometric Function4/1
  Trigonometric Function5/1 -> Product4/1, Product7/3
  Trigonometric Function3/1 -> Product6/1
  theta/1 -> Trigonometric Function3/1, Trigonometric Function2/1
  Trigonometric Function/1 -> Product4/2, Product3/1
  Trigonometric Function1/1 -> Product5/3, Product6/2, Product7/1
  phi/1 -> Trigonometric Function/1, Trigonometric Function1/1
  Add3/1 -> Out1/1
  Trigonometric Function2/1 -> Product5/2, Product7/2
  Product3/1 -> Add3/2
  Product6/1 -> Out3/1
  Product5/1 -> Add4/1
  Trigonometric Function4/1 -> Product5/1, Product3/2
  Product7/1 -> Add3/1
  Product4/1 -> Add4/2
  Add4/1 -> Out2/1

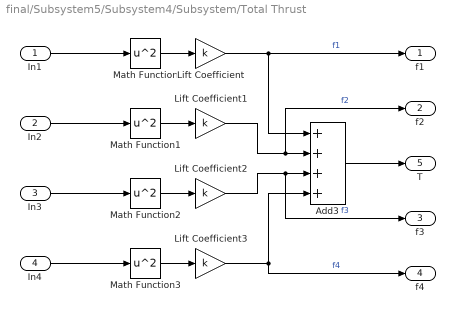
== system final/Subsystem5/Subsystem4/Subsystem/Total Thrust ==
  In1 : Inport
  In2 : Inport  Port=2
  In3 : Inport  Port=3
  In4 : Inport  Port=4
  Add3 : Sum  Inputs=++++
  Lift Coefficient{,1..3} (4 alike) : Gain  Gain=k
  Math Function{,1..3} (4 alike) : Math  Operator=square
  f1 : Outport
  f2 : Outport  Port=2
  f3 : Outport  Port=3
  f4 : Outport  Port=4
  T : Outport  Port=5
  wires:
  Math Function/1 -> Lift Coefficient/1
  Lift Coefficient/1 -> f1/1, Add3/1  "f1"
  Lift Coefficient3/1 -> f4/1, Add3/4  "f4"
  Math Function3/1 -> Lift Coefficient3/1
  Math Function2/1 -> Lift Coefficient2/1
  Lift Coefficient1/1 -> f2/1, Add3/2  "f2"
  Math Function1/1 -> Lift Coefficient1/1
  In4/1 -> Math Function3/1
  Lift Coefficient2/1 -> f3/1, Add3/3  "f3"
  In3/1 -> Math Function2/1
  In2/1 -> Math Function1/1
  In1/1 -> Math Function/1
  Add3/1 -> T/1

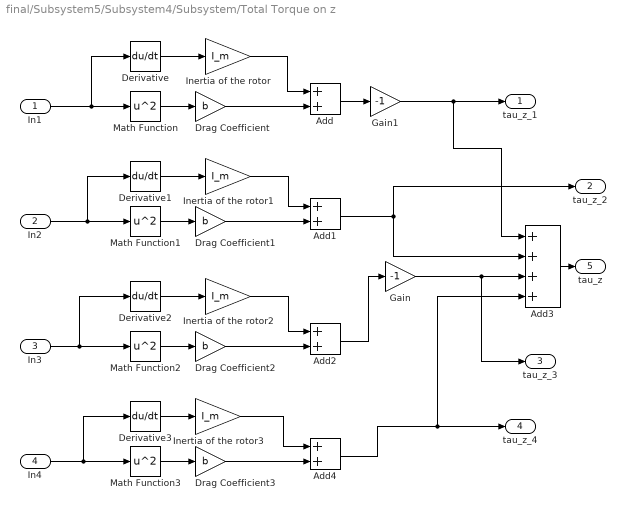
== system final/Subsystem5/Subsystem4/Subsystem/Total Torque on z ==
  In1 : Inport
  In2 : Inport  Port=2
  In3 : Inport  Port=3
  In4 : Inport  Port=4
  Add{,1..2,4} (4 alike) : Sum
  Add3 : Sum  Inputs=++++
  Derivative{,1..3} (4 alike) : Derivative
  Drag Coefficient{,1..3} (4 alike) : Gain  Gain=b
  Gain : Gain  Gain=-1
  Gain1 : Gain  Gain=-1
  Inertia of the rotor{,1..3} (4 alike) : Gain  Gain=I_m
  Math Function{,1..3} (4 alike) : Math  Operator=square
  tau_z_1 : Outport
  tau_z_2 : Outport  Port=2
  tau_z_3 : Outport  Port=3
  tau_z_4 : Outport  Port=4
  tau_z : Outport  Port=5
  wires:
  Math Function/1 -> Drag Coefficient/1
  Math Function3/1 -> Drag Coefficient3/1
  Math Function2/1 -> Drag Coefficient2/1
  Math Function1/1 -> Drag Coefficient1/1
  In4/1 -> Derivative3/1, Math Function3/1
  In2/1 -> Derivative1/1, Math Function1/1
  In1/1 -> Derivative/1, Math Function/1
  Add3/1 -> tau_z/1
  Derivative/1 -> Inertia of the rotor/1
  Drag Coefficient/1 -> Add/2
  Inertia of the rotor/1 -> Add/1
  Derivative1/1 -> Inertia of the rotor1/1
  Drag Coefficient1/1 -> Add1/2
  Inertia of the rotor1/1 -> Add1/1
  In3/1 -> Derivative2/1, Math Function2/1
  Derivative2/1 -> Inertia of the rotor2/1
  Drag Coefficient2/1 -> Add2/2
  Inertia of the rotor2/1 -> Add2/1
  Derivative3/1 -> Inertia of the rotor3/1
  Drag Coefficient3/1 -> Add4/2
  Inertia of the rotor3/1 -> Add4/1
  Add/1 -> Gain1/1
  Add1/1 -> Add3/2, tau_z_2/1
  Add2/1 -> Gain/1
  Add4/1 -> tau_z_4/1, Add3/4
  Gain1/1 -> tau_z_1/1, Add3/1
  Gain/1 -> tau_z_3/1, Add3/3
